simulink library "INT_HLSDem_SelectParameter"  (R2016b)
settings: Solver=VariableStepAuto  StartTime=0.0  StopTime=10.0  RelTol=1e-3
settings Model: Creator=xuxingpei  LastModifiedBy=xuxingpei

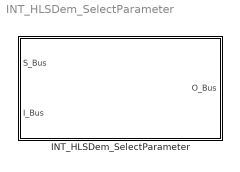
== system INT_HLSDem_SelectParameter ==
  INT_HLSDem_SelectParameter : Subsystem

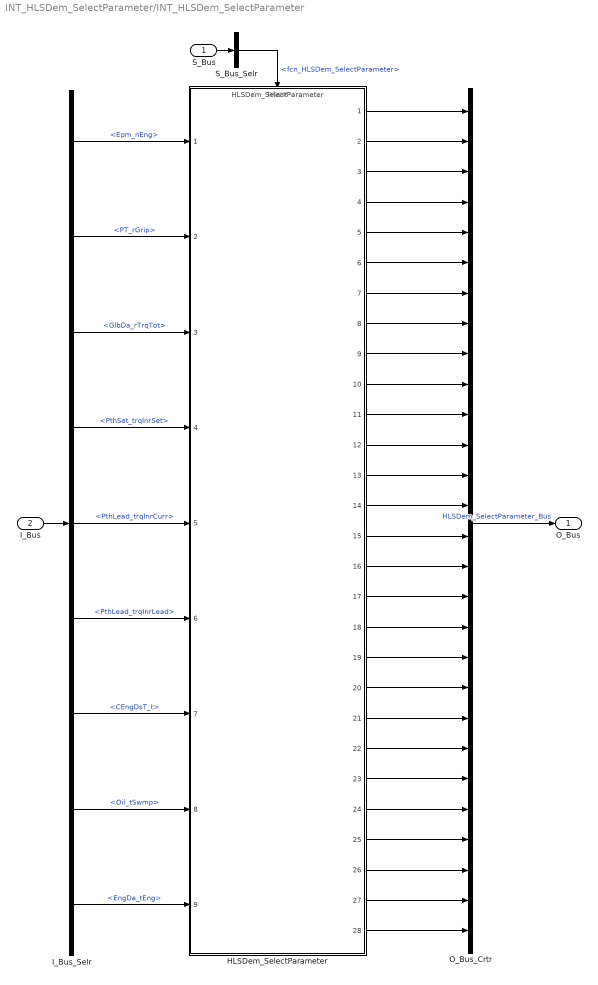
== system INT_HLSDem_SelectParameter/INT_HLSDem_SelectParameter ==
  S_Bus : Inport
  I_Bus : Inport  Port=2
  HLSDem_SelectParameter : ModelReference  ModelNameDialog=HLSDem_SelectParameter  SimulationMode=Normal  ModelReferenceVersion=1.84  TriggerPortName=function  TriggerPortTriggerType=function-call  TriggerPortStatesWhenEnabling=held
  I_Bus_Selr : BusSelector  OutputSignals=Epm_nEng,PT_rGrip,GlbDa_rTrqTot,PthSet_trqInrSet,PthLead_trqInrCurr,PthLead_trqInrLead,CEngDsT_t,Oil_tSwmp,EngDa_tEng
  O_Bus_Crtr : BusCreator  Inputs=28
  S_Bus_Selr : BusSelector  OutputSignals=fcn_HLSDem_SelectParameter
  O_Bus : Outport
  wires:
  S_Bus_Selr/1 -> HLSDem_SelectParameter/Trigger  "<fcn_HLSDem_SelectParameter>"
  S_Bus/1 -> S_Bus_Selr/1
  I_Bus/1 -> I_Bus_Selr/1
  I_Bus_Selr/1 -> HLSDem_SelectParameter/1  "<Epm_nEng>"
  I_Bus_Selr/2 -> HLSDem_SelectParameter/2  "<PT_rGrip>"
  I_Bus_Selr/3 -> HLSDem_SelectParameter/3  "<GlbDa_rTrqTot>"
  I_Bus_Selr/4 -> HLSDem_SelectParameter/4  "<PthSet_trqInrSet>"
  I_Bus_Selr/5 -> HLSDem_SelectParameter/5  "<PthLead_trqInrCurr>"
  I_Bus_Selr/6 -> HLSDem_SelectParameter/6  "<PthLead_trqInrLead>"
  I_Bus_Selr/7 -> HLSDem_SelectParameter/7  "<CEngDsT_t>"
  I_Bus_Selr/8 -> HLSDem_SelectParameter/8  "<Oil_tSwmp>"
  I_Bus_Selr/9 -> HLSDem_SelectParameter/9  "<EngDa_tEng>"
  O_Bus_Crtr/1 -> O_Bus/1  "HLSDem_SelectParameter_Bus"
  HLSDem_SelectParameter/1 -> O_Bus_Crtr/1
  HLSDem_SelectParameter/2 -> O_Bus_Crtr/2
  HLSDem_SelectParameter/3 -> O_Bus_Crtr/3
  HLSDem_SelectParameter/4 -> O_Bus_Crtr/4
  HLSDem_SelectParameter/5 -> O_Bus_Crtr/5
  HLSDem_SelectParameter/6 -> O_Bus_Crtr/6
  HLSDem_SelectParameter/7 -> O_Bus_Crtr/7
  HLSDem_SelectParameter/8 -> O_Bus_Crtr/8
  HLSDem_SelectParameter/9 -> O_Bus_Crtr/9
  HLSDem_SelectParameter/10 -> O_Bus_Crtr/10
  HLSDem_SelectParameter/11 -> O_Bus_Crtr/11
  HLSDem_SelectParameter/12 -> O_Bus_Crtr/12
  HLSDem_SelectParameter/13 -> O_Bus_Crtr/13
  HLSDem_SelectParameter/14 -> O_Bus_Crtr/14
  HLSDem_SelectParameter/15 -> O_Bus_Crtr/15
  HLSDem_SelectParameter/16 -> O_Bus_Crtr/16
  HLSDem_SelectParameter/17 -> O_Bus_Crtr/17
  HLSDem_SelectParameter/18 -> O_Bus_Crtr/18
  HLSDem_SelectParameter/19 -> O_Bus_Crtr/19
  HLSDem_SelectParameter/20 -> O_Bus_Crtr/20
  HLSDem_SelectParameter/21 -> O_Bus_Crtr/21
  HLSDem_SelectParameter/22 -> O_Bus_Crtr/22
  HLSDem_SelectParameter/23 -> O_Bus_Crtr/23
  HLSDem_SelectParameter/24 -> O_Bus_Crtr/24
  HLSDem_SelectParameter/25 -> O_Bus_Crtr/25
  HLSDem_SelectParameter/26 -> O_Bus_Crtr/26
  HLSDem_SelectParameter/27 -> O_Bus_Crtr/27
  HLSDem_SelectParameter/28 -> O_Bus_Crtr/28
